simulink model "Wk2_Q1_PID"  (R2022b)
settings: Solver=VariableStepAuto  StartTime=0.0  StopTime=10.0  RelTol=1e-3
values from neighbouring files (symbols this model uses):
  kd = 0.9    [Wk2_Q1.m]
  ki = 6    [Wk2_Q1.m]
  kp = 8    [Wk2_Q1.m]
settings Model: Creator=zd012  LastModifiedBy=zd012

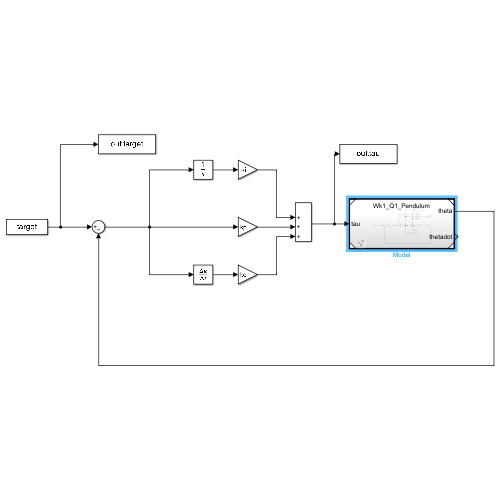
[thumbnail: Simulink's stored preview of the top-level diagram]
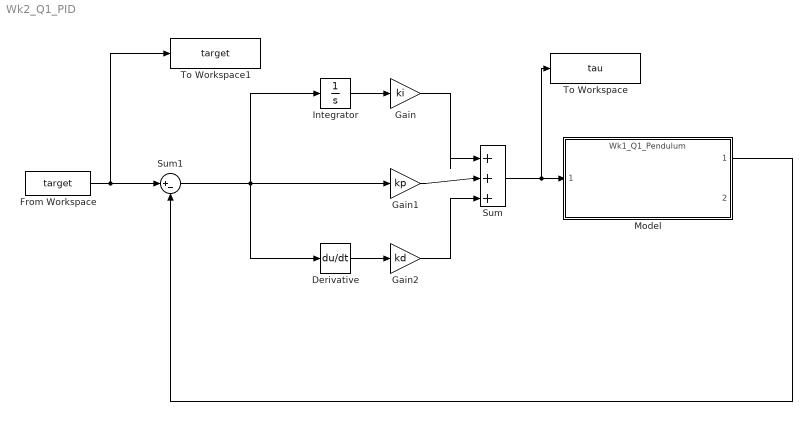
== system Wk2_Q1_PID ==
  Derivative : Derivative
  From Workspace : FromWorkspace  VariableName=target
  Gain : Gain  Gain=ki
  Gain1 : Gain  Gain=kp
  Gain2 : Gain  Gain=kd
  Integrator : Integrator
  Model : ModelReference  ModelNameDialog=Wk1_Q1_Pendulum  SimulationMode=Normal  ModelReferenceVersion=4.6
  Sum : Sum  Inputs=|+++
  Sum1 : Sum  Inputs=|+-
  To Workspace : ToWorkspace  VariableName=tau  SampleTime=-1
      settings: Save2DSignal=2-D array (concatenate along first dimension)
  To Workspace1 : ToWorkspace  VariableName=target  SampleTime=-1
      settings: Save2DSignal=2-D array (concatenate along first dimension)
  wires:
  Integrator/1 -> Gain/1
  Gain/1 -> Sum/1
  Gain1/1 -> Sum/2
  Gain2/1 -> Sum/3
  Sum/1 -> To Workspace/1, Model/1
  Model/1 -> Sum1/2
  From Workspace/1 -> To Workspace1/1, Sum1/1
  Sum1/1 -> Derivative/1, Gain1/1, Integrator/1
  Derivative/1 -> Gain2/1
